simulink model "hvac_maborrelli_singapur_nzones_T2"  (R2021a)
settings: Solver=ode45  StartTime=0.0  StopTime=Inf  FixedStep=2  RelTol=1e-3  EnableMultiTasking=on
undefined symbols (not defined in the file): beta, ci, high, low, params, paramsnz, rl, scale, Ts, Ts2
libraries: dspmathops x3, simulink x2, rllib x1
settings Model: Creator=User  LastModifiedBy=Richi
settings SolverCC: AlgebraicLoopSolver=TrustRegion
settings DataIOCC: LimitDataPoints=on  SaveFormat=Array  SignalLoggingSaveFormat=ModelDataLogs
settings OptimizationCC: LifeSpan=inf
settings DebuggingCC: SolverPrmCheckMsg=warning  MultiTaskDSMMsg=warning  MultiTaskCondExecSysMsg=none  MultiTaskRateTransMsg=warning  StrictBusMsg=ErrorOnBusTreatedAsVector  SFUnexpectedBacktrackingDiag=warning  SFNoUnconditionalDefaultTransitionDiag=warning  SFExecutionAtInitializationDiag=none  SFMachineParentedDataDiag=warning  ArithmeticOperatorsInVariantConditions=warning
settings HardwareCC: ProdBitPerPointer=32  ProdBitPerSizeT=32  ProdBitPerPtrDiffT=32  ProdLargestAtomicFloat=None  ProdIntDivRoundTo=Undefined  ProdEndianess=Unspecified  ProdWordSize=32  ProdHWDeviceType=32-bit Generic
settings ModelReferenceCC: PropagateSignalLabelsOutOfModel=off
settings SFSimCC: SimUseLocalCustomCode=off  CustomCodeUndefinedFunction=UseInterfaceOnly
settings RTWCC: RTWUseLocalCustomCode=off
settings CodeAppCC: StateflowObjectComments=on
settings GRTTargetCC: TargetLangStandard=C89/C90 (ANSI)
settings ConfigComp: CovMetricSettings=dw  CovSaveCumulativeToWorkspaceVar=on  CovSaveSingleToWorkspaceVar=on  CovExternalEMLEnable=off

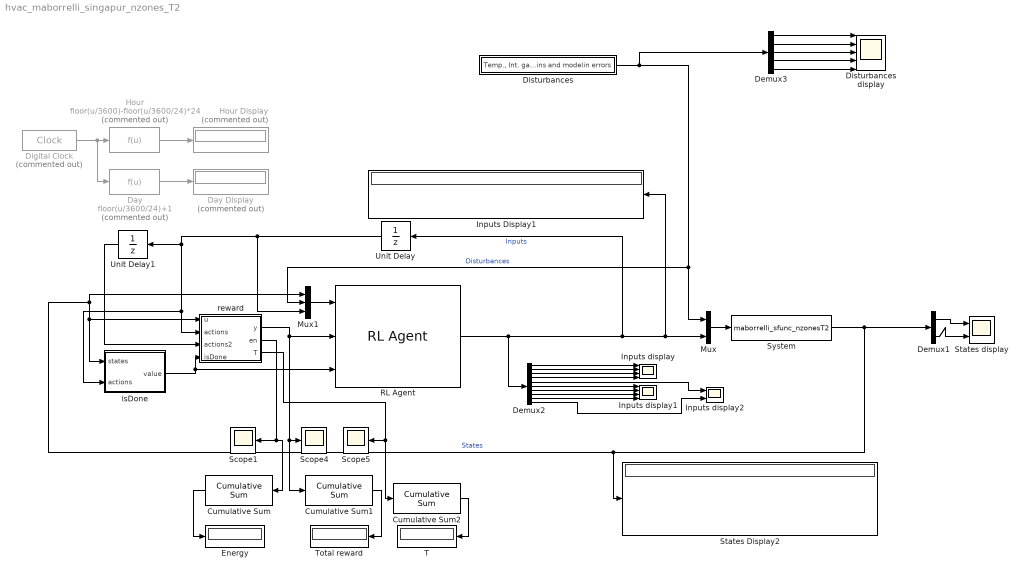
== system hvac_maborrelli_singapur_nzones_T2 ==
  Cumulative Sum : dspmathops/Cumulative Sum  dim=Channels (running sum)  InputProcessing=Columns as channels (frame based)  reset_popup=None  roundingMode=Floor  overflowMode=off  outputDataTypeStr=Inherit: Same as accumulator  outputMin=[]  outputMax=[]  outputLastDataTypeStr=Inherit: Same as accumulator
  Cumulative Sum1 : dspmathops/Cumulative Sum  dim=Channels (running sum)  InputProcessing=Columns as channels (frame based)  reset_popup=None  roundingMode=Floor  overflowMode=off  outputDataTypeStr=Inherit: Same as accumulator  outputMin=[]  outputMax=[]  outputLastDataTypeStr=Inherit: Same as accumulator
  Cumulative Sum2 : dspmathops/Cumulative Sum  dim=Channels (running sum)  InputProcessing=Columns as channels (frame based)  reset_popup=None  roundingMode=Floor  overflowMode=off  outputDataTypeStr=Inherit: Same as accumulator  outputMin=[]  outputMax=[]  outputLastDataTypeStr=Inherit: Same as accumulator
  Day : Fcn  Commented=on  Expr=floor(u/3600/24)+1  SampleTime=1800
  Day Display : Display  Commented=on
  Demux1 : Demux  Outputs=2
  Demux2 : Demux  Outputs=10
  Demux3 : Demux  Outputs=5
  Digital Clock : DigitalClock  Commented=on  SampleTime=60
  Disturbances : Subsystem  TreatAsAtomicUnit=on
  Disturbances display : Scope  NumInputPorts=5
  Energy : Display
  Hour : Fcn  Commented=on  Expr=floor(u/3600)-floor(u/3600/24)*24  SampleTime=1800
  Hour Display : Display  Commented=on
  Inputs Display1 : Display
  Inputs display : Scope  NumInputPorts=4
  Inputs display1 : Scope  NumInputPorts=4
  Inputs display2 : Scope  NumInputPorts=2
  Mux : Mux  Inputs=2
  Mux1 : Mux  Inputs=3
  RL Agent : rllib/RL Agent  Agent=rl.util.PolicyInstance.get('hvac_maborrelli_singapur_nzones_T/RL Agent')  ExternalActionAsInput=off  ProvideCumRwd=off  TreatAsDirectFeedthrough=on
  Scope1 : Scope
  Scope4 : Scope
  Scope5 : Scope
  States Display2 : Display
  States display : Scope  NumInputPorts=2
  System : S-Function  FunctionName=maborrelli_sfunc_nzonesT2  Parameters=ci,paramsnz,Ts  SFunctionDeploymentMode=off  EnableBusSupport=off
  T : Display
  Total reward : Display
  Unit Delay : UnitDelay  SampleTime=Ts2  HasFrameUpgradeWarning=on
  Unit Delay1 : UnitDelay  SampleTime=Ts2  HasFrameUpgradeWarning=on
  isDone : MATLAB Function  TreatAsAtomicUnit=on
  reward : MATLAB Function  TreatAsAtomicUnit=on
  wires:
  Mux/1 -> System/1
  System/1 -> Demux1/1, States Display2/1, Mux1/1, isDone/1(states), reward/1(u)  "States"
  RL Agent/1 -> Unit Delay/1, Mux/2, Inputs Display1/1, Demux2/1  "Inputs"
  Hour/1 -> Hour Display/1
  Digital Clock/1 -> Day/1, Hour/1
  Day/1 -> Day Display/1
  Demux1/1 -> States display/1
  Demux1/2 -> States display/2
  Demux2/1 -> Inputs display/1
  Demux2/2 -> Inputs display/2
  Demux2/3 -> Inputs display/3
  Demux2/4 -> Inputs display/4
  isDone/1(value) -> reward/4(isDone), RL Agent/3
  Mux1/1 -> RL Agent/1
  Unit Delay/1 -> Mux1/3, Unit Delay1/1, isDone/2(actions), reward/2(actions)
  Disturbances/1("Temp., Int. gains and modelin errors") -> Mux1/2, Mux/1, Demux3/1  "Disturbances"
  Demux3/1 -> Disturbances display/1
  Cumulative Sum/1 -> Energy/1
  Cumulative Sum2/1 -> T/1
  reward/1(y) -> Cumulative Sum1/1, Scope4/1, RL Agent/2
  reward/3(T) -> Cumulative Sum2/1, Scope5/1
  Cumulative Sum1/1 -> Total reward/1
  reward/2(en) -> Cumulative Sum/1, Scope1/1
  Demux3/2 -> Disturbances display/2
  Demux3/3 -> Disturbances display/3
  Demux3/4 -> Disturbances display/4
  Demux3/5 -> Disturbances display/5
  Demux2/6 -> Inputs display1/1
  Demux2/8 -> Inputs display1/3
  Demux2/7 -> Inputs display1/2
  Demux2/9 -> Inputs display1/4
  Demux2/5 -> Inputs display2/1
  Demux2/10 -> Inputs display2/2
  Unit Delay1/1 -> reward/3(actions2)

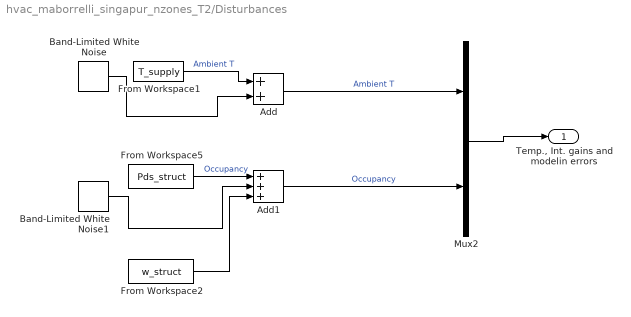
== system hvac_maborrelli_singapur_nzones_T2/Disturbances ==
  Add : Sum
  Add1 : Sum  Inputs=+++
  Band-Limited White Noise : simulink/Sources/Band-Limited White Noise  Cov=0  Ts=Ts2  seed=[23341]
  Band-Limited White Noise1 : simulink/Sources/Band-Limited White Noise  Cov=0  Ts=Ts2  seed=[23341]
  From Workspace1 : FromWorkspace  VariableName=T_supply  OutDataTypeStr=double  SampleTime=Ts  ZeroCross=off
  From Workspace2 : FromWorkspace  VariableName=w_struct  OutDataTypeStr=double  SampleTime=Ts  ZeroCross=off
  From Workspace5 : FromWorkspace  VariableName=Pds_struct  OutDataTypeStr=double  SampleTime=Ts  ZeroCross=off
  Mux2 : Mux  Inputs=2
  "Temp., Int. gains and modelin errors" : Outport
  wires:
  Add1/1 -> Mux2/2  "Occupancy"
  From Workspace1/1 -> Add/1  "Ambient T"
  Band-Limited White Noise/1 -> Add/2
  Add/1 -> Mux2/1  "Ambient T"
  From Workspace5/1 -> Add1/1  "Occupancy"
  Band-Limited White Noise1/1 -> Add1/2
  From Workspace2/1 -> Add1/3
  Mux2/1 -> "Temp., Int. gains and modelin errors"/1

== matlab function hvac_maborrelli_singapur_nzones_T2/isDone ==
  data: states input; value output; actions input
function value = isDone(states,actions)
 low = -0;
 max = 50;
 value = 0; 
 %disp(length(block.InputPort(1).Data))
 for i=1:length(states)
     %disp(i)
     if sum(actions(2:5)) > 5
        value = 1;
        break
     end
     if i <=4
        aux = states(i);
        if (aux < low || aux > max) 
            %disp(abs(aux - low))
            value = 1;
            break
        end
     elseif i>=9 && i<=12
        if states(i)>(3200*1e-6)
            value = 1;
            break
        end
     end
 end

== matlab function hvac_maborrelli_singapur_nzones_T2/reward ==
  data: u input; y output; actions input; actions2 input; isDone input; en output; T output; low parameter; high parameter; beta parameter; params parameter; scale parameter
function [y, en, T] = reward(u ,  actions, actions2 , isDone, low, high, beta, params, scale)
 reward = 0;
 cp = params.cp;
 eta = params.eta;
 kf = params.kf;
 eta_h = params.eta_h;
 nz = 4;
 ms = actions(1:nz);
 Dt = actions(nz+1);
 Dth = actions(nz+2:2*nz+1);
 delta = actions(2*nz + 2);
 ms0 = actions2(1:nz);
 Dt0 = actions2(nz+1);
 Dth0 = actions2(nz+2:2*nz+1);
 delta0 = actions2(2*nz + 2);
 T_in = u(1:nz);
 %Se inician las metricas
 T = 0;
 if sum(ms) > 5
     reward = -5000;
 end
 %Añadir energía:
 %Energía utilizada por ventilador
 e = (kf*sum((ms).^2))/1000;
 %Energía por enfriar
 e = e + ((-cp/eta)*sum(ms)*(Dt))/1000;
 if abs(Dt0 - Dt) > 0.5*scale(nz+1)
     reward = reward - 10;
 end
 if abs(delta0 - delta) > 0.5*scale(2*nz + 2)
     reward = reward - 100;
 end
 for i=1:nz
     if abs(ms(i) - ms0(i)) > 0.5*scale(1)
        reward = reward - 100;
     end
     %Se aplica la penalización por energía al usar la calefacción
     if Dth(i) ~= 0
         e = e + ((cp/eta_h)*ms(i)*(Dth(i) - Dt))/1000;
     end
     %Se penaliza si hay calefacción pero no flujo de aire.
     if ms(i) == 0 && Dth(i)~=0
         reward = reward - 10;
     end
     %Se penaliza si hay enfriamiento pero no flujo de aire.
     if ms(i) == 0 && Dt~=0
         reward = reward - 0.5;
     end
     %Se penaliza romper las restricciones de temperatura.
     aux = T_in(i);
     if (aux < low || aux > high)
        T = T + 0.5*(min(abs(aux - low), abs(aux - high))+ (min( abs(aux - low), abs(aux - high)))^2);
        %reward = reward - T;
     end
     %Entregar bonificación por estar en el estado
     %if (aux >= low && aux <= high)
     %    reward = reward + 1;
     %end
 %Se aplica el peso a la energía
 reward = reward - beta*e; 
 %Se aplica la penalización por estado
 reward = reward - T;
 en = e;
 end
 
 if isDone
     reward = -8000;
 end
y = reward;
